simulink model "Assignment1"  (R2014a)
settings: Solver=FixedStepDiscrete  StartTime=0.0  StopTime=100000  FixedStep=1  RelTol=1e-3
libraries: simulink x1, hdlsllib x1
settings Model: Creator=vu.du  LastModifiedBy=vu.du

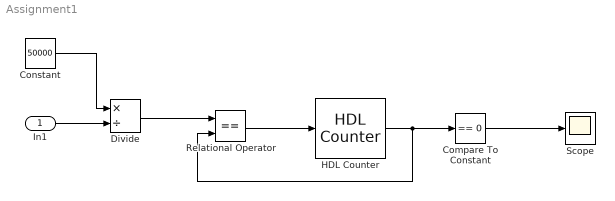
== system Assignment1 ==
  In1 : Inport
  Compare To Constant : simulink/Logic and Bit Operations/Compare To Constant  relop===  const=0  OutDataTypeStr=boolean
  Constant : Constant  Value=50000  OutDataTypeStr=int32
  Divide : Product  Inputs=*/  OutDataTypeStr=int32  SaturateOnIntegerOverflow=on  RndMeth=Zero
  HDL Counter : hdlsllib/HDL Operations/HDL Counter  CountType=Free running  CountInit=0  CountStep=1  CountMax=100  CountFromType=Initial value  CountFrom=0  CountResetPort=on  CountLoadPort=off  CountEnbPort=off  CountDirPort=off  CountDataType=Unsigned  CountWordLen=32  CountFracLen=0  CountSampTime=1
  Relational Operator : RelationalOperator  Operator===  OutDataTypeStr=boolean
  Scope : Scope
  wires:
  HDL Counter/1 -> Relational Operator/2, Compare To Constant/1
  Compare To Constant/1 -> Scope/1
  In1/1 -> Divide/2
  Constant/1 -> Divide/1
  Divide/1 -> Relational Operator/1
  Relational Operator/1 -> HDL Counter/1
